simulink model "HandExosThumbRAL_EMG"  (R2013a)
settings: Solver=FixedStepDiscrete  StartTime=0.0  StopTime=inf  FixedStep=1/256  RelTol=1e-3
undefined symbols (not defined in the file or in its folder): currentCFG_EMGTest_UB, serial, UB
libraries: etargetslib x6, instrumentlib x6, dspnetwork x2, xpcutilitieslib x1, gUSBamplib x1
settings Model: Creator=mine  LastModifiedBy=BCI-USER

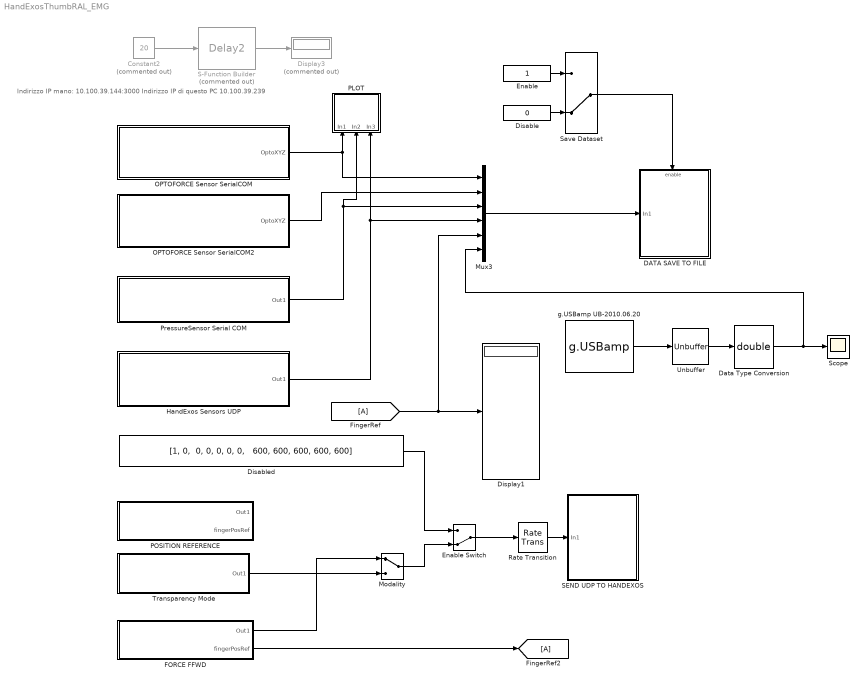
== system HandExosThumbRAL_EMG ==
  note: Indirizzo IP mano: 10.100.39.144:3000
      | Indirizzo IP di questo PC 10.100.39.239
  Constant2 : Constant  Commented=on  Value=20  OutDataTypeStr=uint32  SampleTime=-1
  DATA SAVE TO FILE : Subsystem  TreatAsAtomicUnit=on
  Data Type Conversion : DataTypeConversion  OutDataTypeStr=double
  Disable : Constant  Value=0  OutDataTypeStr=double  SampleTime=-1
  Disabled : Constant  Value="[1, 0,  0, 0, 0, 0, 0,   600, 600, 600, 600, 600]"  OutDataTypeStr=double  SampleTime=-1
  Display1 : Display
  Display3 : Display  Commented=on
  Enable : Constant  OutDataTypeStr=double  SampleTime=-1
  Enable Switch : ManualSwitch  CurrentSetting=0
  FORCE FFWD : Subsystem
  HandExos Sensors UDP : Subsystem
  "Modality " : ManualSwitch
  Mux3 : Mux  Inputs=6
  OPTOFORCE Sensor SerialCOM : Subsystem
  OPTOFORCE Sensor SerialCOM2 : Subsystem
  PLOT : Subsystem
  POSITION REFERENCE : Subsystem
  PressureSensor Serial COM : Subsystem
  Rate Transition : RateTransition
  S-Function Builder : S-Function  Commented=on  InitFcn=try, set_param(gcb,'FunctionName','Delay2'), end  FunctionName=Delay2  SFunctionModules=Delay2_wrapper  EnableBusSupport=off  mask(S-Function Builder){}
      mask help: Simulink:masks:SFunctionBuilder_MD
      mask init:
      | val = [[.9  0.75 0.75 1 1 .9 .9 1]',[1 1 0.75 0.75 .9 .9 1 .9]'];try , sys = get_param(gcb,'SfunBuilderFcnName');if isempty(sys), sys = get_param(gcb,'FunctionName'); end,catch, sys = get_param(gcb,'FunctionName'); end
      settings: CopyFcn=set_param(gcbh,'LinkStatus','none')  PreSaveFcn=try, set_param(gcb,'FunctionName','Delay2'), end  OpenFcn=sfunctionwizard(gcbh)
      mask Display: plot(val(:,1),val(:,2)),disp(sys), port_label('input',1,'u0'), port_label('output',1,'y0')
  SEND UDP TO HANDEXOS : Subsystem  TreatAsAtomicUnit=on  SystemSampleTime=4/256
  Save Dataset : ManualSwitch  CurrentSetting=0
  Scope : Scope
      settings: TimeRange=8  YMin=-225  YMax=200  SaveName=ScopeData3
  Transparency Mode : Subsystem
  Unbuffer : Unbuffer  SampleBasedProcessing=Same as frame based
  g.USBamp UB-2010.06.20 : gUSBamplib/g.USBamp  cfg=currentCFG_EMGTest_UB-2010.06.20.cfg  snr=UB-2010.06.20
  wires:
  Constant2/1 -> S-Function Builder/1
  S-Function Builder/1 -> Display3/1
  Disabled/1 -> Enable Switch/1
  Disable/1 -> Save Dataset/2
  Enable/1 -> Save Dataset/1
  Save Dataset/1 -> DATA SAVE TO FILE/Enable
  OPTOFORCE Sensor SerialCOM/1(OptoXYZ) -> PLOT/1(In1), Mux3/1
  Mux3/1 -> DATA SAVE TO FILE/1(In1)
  Transparency Mode/1(Out1) -> "Modality "/2
  Enable Switch/1 -> Rate Transition/1
  HandExos Sensors UDP/1(Out1) -> Mux3/4, PLOT/3(In3)
  [A] -> Mux3/5, Display1/1
  PressureSensor Serial COM/1(Out1) -> PLOT/2(In2), Mux3/3
  "Modality "/1 -> Enable Switch/2
  OPTOFORCE Sensor SerialCOM2/1(OptoXYZ) -> Mux3/2
  FORCE FFWD/1(Out1) -> "Modality "/1
  FORCE FFWD/2(fingerPosRef) -> [A]
  g.USBamp UB-2010.06.20/1 -> Unbuffer/1
  Unbuffer/1 -> Data Type Conversion/1
  Rate Transition/1 -> SEND UDP TO HANDEXOS/1(In1)
  Data Type Conversion/1 -> Mux3/6, Scope/1

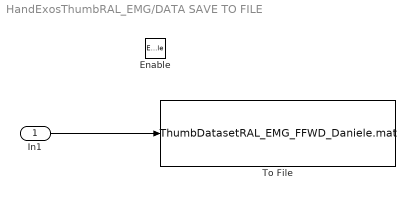
== system HandExosThumbRAL_EMG/DATA SAVE TO FILE ==
  In1 : Inport
  Enable : EnablePort
  To File : ToFile  Filename=ThumbDatasetRAL_EMG_FFWD_Daniele.mat  MatrixName=data
  wires:
  In1/1 -> To File/1

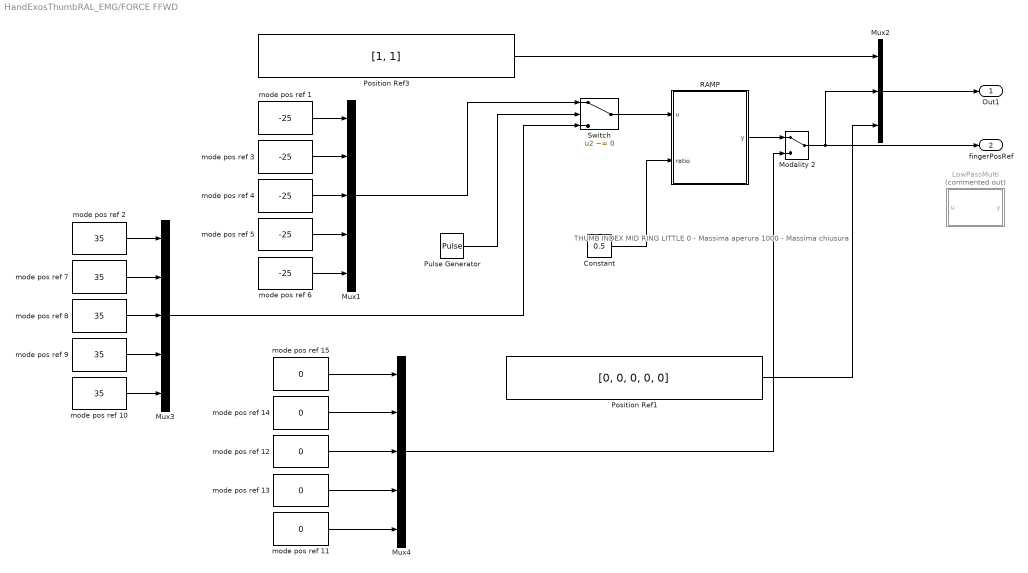
== system HandExosThumbRAL_EMG/FORCE FFWD ==
  note: THUMB
      | INDEX
      | MID
      | RING
      | LITTLE
      |
      | 0 - Massima aperura
      | 1000 - Massima chiusura
  Constant : Constant  Value=0.5
  LowPassMulti : MATLAB Function  Commented=on  TreatAsAtomicUnit=on
  Modality 2 : ManualSwitch
  Mux1 : Mux  Inputs=5
  Mux2 : Mux  Inputs=3
  Mux3 : Mux  Inputs=5
  Mux4 : Mux  Inputs=5
  Position Ref1 : Constant  Value=[0, 0, 0, 0, 0]  OutDataTypeStr=double  SampleTime=-1
  Position Ref3 : Constant  Value=[1, 1]  OutDataTypeStr=double  SampleTime=-1
  Pulse Generator : DiscretePulseGenerator  PulseType=Time based  Period=10  PulseWidth=50
  RAMP : MATLAB Function  TreatAsAtomicUnit=on
  Switch : Switch  Criteria=u2 ~= 0
  mode pos ref {1,3..6} (5 alike) : Constant  Value=-25  OutDataTypeStr=double  SampleTime=-1
  mode pos ref {2,7..10} (5 alike) : Constant  Value=35  OutDataTypeStr=double  SampleTime=-1
  mode pos ref {11..15} (5 alike) : Constant  Value=0  OutDataTypeStr=double  SampleTime=-1
  Out1 : Outport
  fingerPosRef : Outport  Port=2
  wires:
  Mux2/1 -> Out1/1
  mode pos ref 1/1 -> Mux1/1
  mode pos ref 6/1 -> Mux1/5
  mode pos ref 5/1 -> Mux1/4
  mode pos ref 4/1 -> Mux1/3
  mode pos ref 3/1 -> Mux1/2
  Position Ref3/1 -> Mux2/1
  mode pos ref 10/1 -> Mux3/5
  mode pos ref 9/1 -> Mux3/4
  mode pos ref 8/1 -> Mux3/3
  mode pos ref 7/1 -> Mux3/2
  mode pos ref 2/1 -> Mux3/1
  mode pos ref 14/1 -> Mux4/2
  mode pos ref 13/1 -> Mux4/4
  mode pos ref 12/1 -> Mux4/3
  mode pos ref 11/1 -> Mux4/5
  Constant/1 -> RAMP/2(ratio)
  Mux1/1 -> Switch/1
  Mux3/1 -> Switch/3
  Pulse Generator/1 -> Switch/2
  mode pos ref 15/1 -> Mux4/1
  RAMP/1(y) -> Modality 2/1
  Modality 2/1 -> Mux2/2, fingerPosRef/1
  Mux4/1 -> Modality 2/2
  Switch/1 -> RAMP/1(u)
  Position Ref1/1 -> Mux2/3

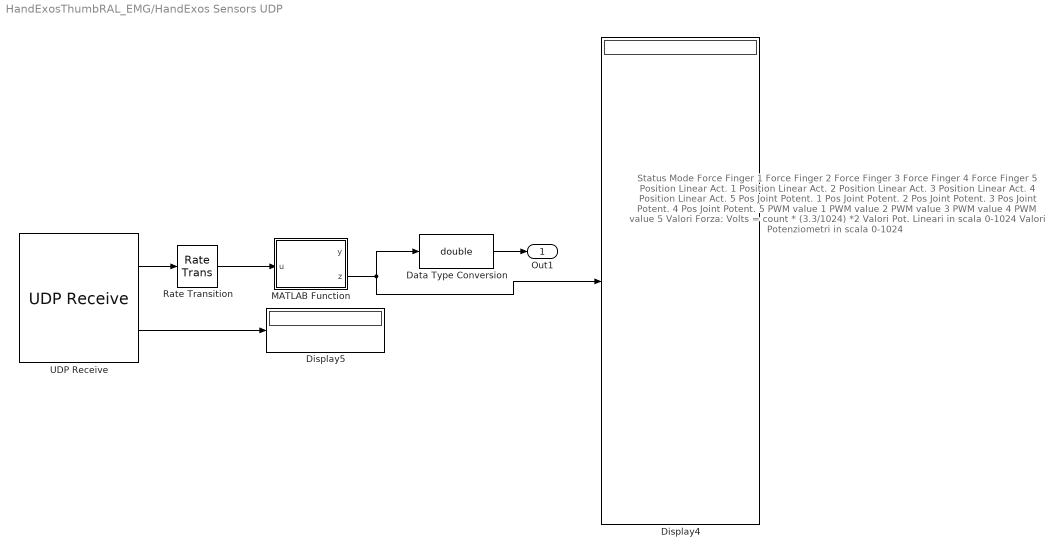
== system HandExosThumbRAL_EMG/HandExos Sensors UDP ==
  note: Status
      | Mode
      | Force Finger 1
      | Force Finger 2
      | Force Finger 3
      | Force Finger 4
      | Force Finger 5
      | Position Linear Act. 1
      | Position Linear Act. 2
      | Position Linear Act. 3
      | Position Linear Act. 4
      | Position Linear Act. 5
      | Pos Joint Potent. 1
      | Pos Joint Potent. 2
      | Pos Joint Potent. 3
      | Pos Joint Potent. 4
      | Pos Joint Potent. 5
      | PWM value 1
      | PWM value 2
      | PWM value 3
      | PWM value 4
      | PWM value 5
      |
      | Valori Forza:    Volts = count * (3.3/1024) *2
      | Valori Pot. Lineari in scala 0-1024
      | Valori Potenziometri in scala 0-1024
  Data Type Conversion : DataTypeConversion  OutDataTypeStr=double
  Display4 : Display
  Display5 : Display
  MATLAB Function : MATLAB Function  TreatAsAtomicUnit=on
  Rate Transition : RateTransition
  UDP Receive : dspnetwork/UDP Receive  localURL='0.0.0.0'  localPort=12001  remoteURL='10.100.39.144'  remotePort=-1  recvBufferSize=73  dims=22  signalDatatype=single  isVarSize=off  showBlockingTime=off  blockingTime=0  sampletime=4/256
  Out1 : Outport
  wires:
  MATLAB Function/2(z) -> Data Type Conversion/1, Display4/1
  UDP Receive/1 -> Rate Transition/1
  UDP Receive/2 -> Display5/1
  Data Type Conversion/1 -> Out1/1
  Rate Transition/1 -> MATLAB Function/1(u)

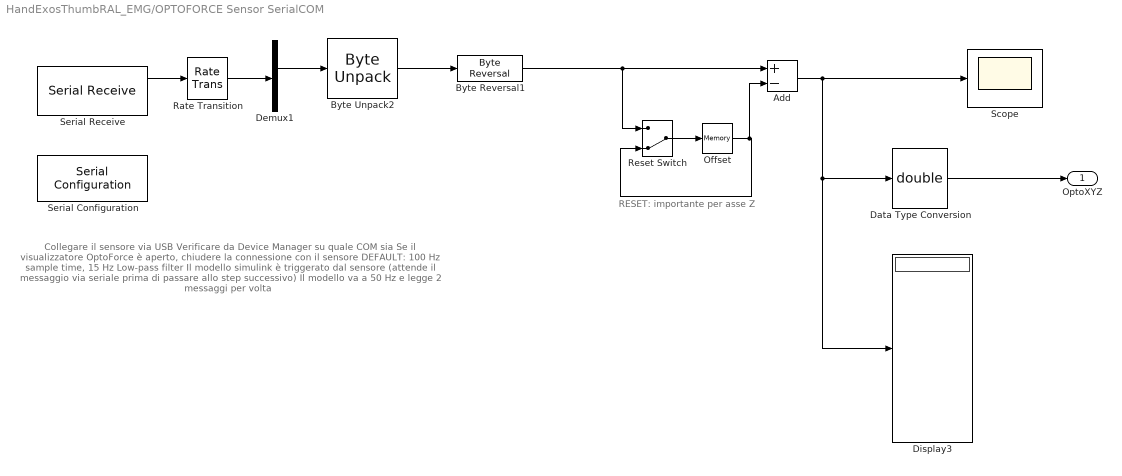
== system HandExosThumbRAL_EMG/OPTOFORCE Sensor SerialCOM ==
  note: RESET: importante per asse Z
  note: Collegare il sensore via USB
      | Verificare da Device Manager su quale COM sia
      | Se il visualizzatore OptoForce è aperto, chiudere la connessione con il sensore
      |
      | DEFAULT: 100 Hz sample time, 15 Hz Low-pass filter
      |
      | Il modello simulink è triggerato dal sensore
      | (attende il messaggio via seriale prima di passare allo step successivo)
      | Il modello va a 50 Hz e legge 2 messaggi per volta
  Add : Sum  Inputs=+-
  Byte Reversal1 : etargetslib/Byte Reversal  numInp=1
  Byte Unpack2 : etargetslib/Byte Unpack  dimensions={3}  datatypes={'int16'}  byteAlign=1
  Data Type Conversion : DataTypeConversion  OutDataTypeStr=double
  Demux1 : Demux  Outputs="[3 6 20  29]"
  Display3 : Display
  Offset : Memory  X0=[0 0 32460]
  Rate Transition : RateTransition
  Reset Switch : ManualSwitch  CurrentSetting=0
  Scope : Scope
      settings: YMin=-800  YMax=1100
  Serial Configuration : instrumentlib/Serial Configuration  Priority=-200000  ComPortMenu=<Please select a port...>  ComPort=COM14  ObjConstructor=serial('COM14');  BaudRate=115200  DataBits=8  Parity=none  StopBits=1  FlowControl=none  Timeout=5  ByteOrder=LittleEndian
  Serial Receive : instrumentlib/Serial Receive  ComPortMenu=COM14  ComPort=COM14  ObjConstructor=serial('COM14');  Terminator=<none>  DataSize="[58   1]"  DataType=uint8  EnableBlockingMode=off  ActionDataUnavailable=Output last received value  CustomValue=0  SampleTime=4/256
  OptoXYZ : Outport
  wires:
  Demux1/2 -> Byte Unpack2/1
  Byte Unpack2/1 -> Byte Reversal1/1
  Reset Switch/1 -> Offset/1
  Offset/1 -> Reset Switch/2, Add/2
  Serial Receive/1 -> Rate Transition/1
  Data Type Conversion/1 -> OptoXYZ/1
  Add/1 -> Display3/1, Data Type Conversion/1, Scope/1
  Byte Reversal1/1 -> Reset Switch/1, Add/1
  Rate Transition/1 -> Demux1/1

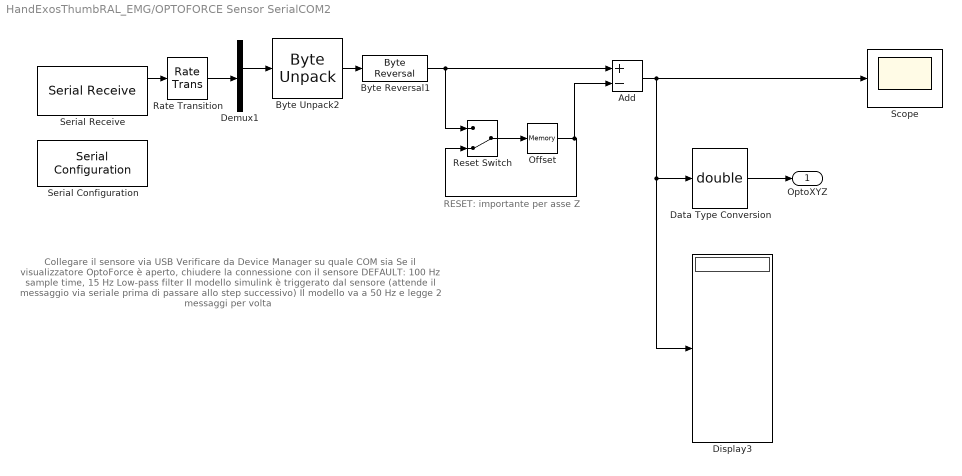
== system HandExosThumbRAL_EMG/OPTOFORCE Sensor SerialCOM2 ==
  note: RESET: importante per asse Z
  note: Collegare il sensore via USB
      | Verificare da Device Manager su quale COM sia
      | Se il visualizzatore OptoForce è aperto, chiudere la connessione con il sensore
      |
      | DEFAULT: 100 Hz sample time, 15 Hz Low-pass filter
      |
      | Il modello simulink è triggerato dal sensore
      | (attende il messaggio via seriale prima di passare allo step successivo)
      | Il modello va a 50 Hz e legge 2 messaggi per volta
  Add : Sum  Inputs=+-
  Byte Reversal1 : etargetslib/Byte Reversal  numInp=1
  Byte Unpack2 : etargetslib/Byte Unpack  dimensions={3}  datatypes={'int16'}  byteAlign=1
  Data Type Conversion : DataTypeConversion  OutDataTypeStr=double
  Demux1 : Demux  Outputs="[3 6 20  29]"
  Display3 : Display
  Offset : Memory  X0=[0 0 32460]
  Rate Transition : RateTransition
  Reset Switch : ManualSwitch  CurrentSetting=0
  Scope : Scope
      settings: YMin=-300  YMax=1200
  Serial Configuration : instrumentlib/Serial Configuration  Priority=-200000  ComPortMenu=COM24  ComPort=COM24  ObjConstructor=serial('COM24');  BaudRate=115200  DataBits=8  Parity=none  StopBits=1  FlowControl=none  Timeout=5  ByteOrder=LittleEndian
  Serial Receive : instrumentlib/Serial Receive  ComPortMenu=COM24  ComPort=COM24  ObjConstructor=serial('COM24');  Terminator=<none>  DataSize="[58   1]"  DataType=uint8  EnableBlockingMode=off  ActionDataUnavailable=Output last received value  CustomValue=0  SampleTime=4/256
  OptoXYZ : Outport
  wires:
  Demux1/2 -> Byte Unpack2/1
  Byte Reversal1/1 -> Reset Switch/1, Add/1
  Byte Unpack2/1 -> Byte Reversal1/1
  Reset Switch/1 -> Offset/1
  Add/1 -> Display3/1, Data Type Conversion/1, Scope/1
  Serial Receive/1 -> Rate Transition/1
  Offset/1 -> Reset Switch/2, Add/2
  Data Type Conversion/1 -> OptoXYZ/1
  Rate Transition/1 -> Demux1/1

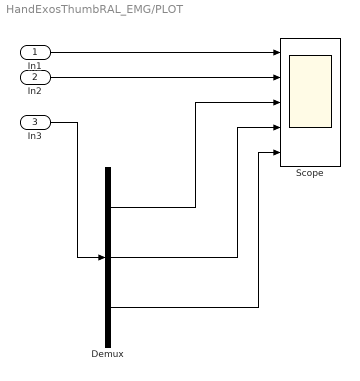
== system HandExosThumbRAL_EMG/PLOT ==
  In1 : Inport
  In2 : Inport  Port=2
  In3 : Inport  Port=3
  Demux : Demux  Outputs=[2 1 4 1 9 1 4]
  Scope : Scope  NumInputPorts=5
      settings: YMin=-1000~237000~32.5~0~-30  YMax=5000~244000~60~350~40  SaveName=ScopeData2
  wires:
  In1/1 -> Scope/1
  In2/1 -> Scope/2
  In3/1 -> Demux/1
  Demux/2 -> Scope/3
  Demux/4 -> Scope/4
  Demux/6 -> Scope/5

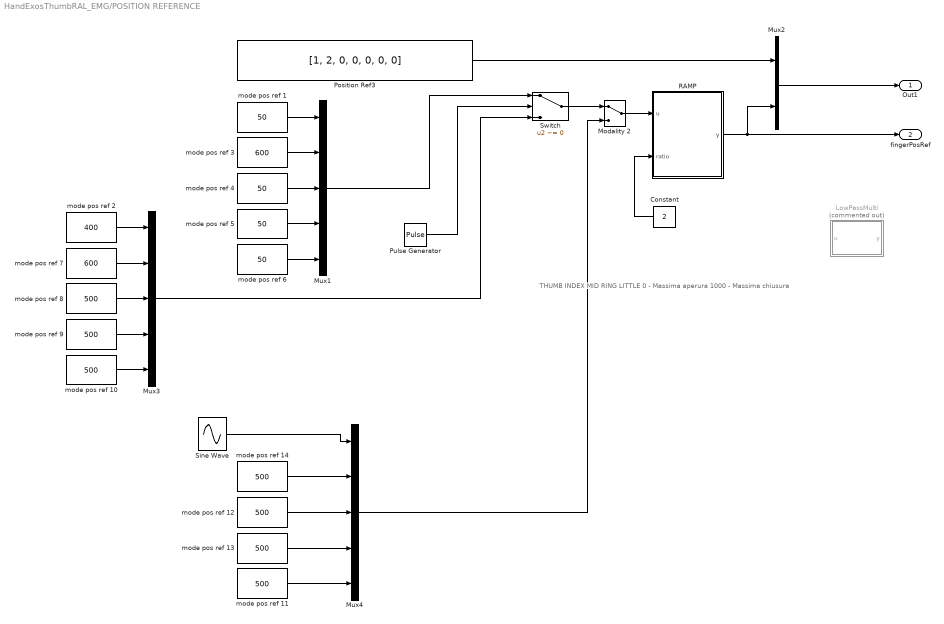
== system HandExosThumbRAL_EMG/POSITION REFERENCE ==
  note: THUMB
      | INDEX
      | MID
      | RING
      | LITTLE
      |
      | 0 - Massima aperura
      | 1000 - Massima chiusura
  Constant : Constant  Value=2
  LowPassMulti : MATLAB Function  Commented=on  TreatAsAtomicUnit=on
  Modality 2 : ManualSwitch
  Mux1 : Mux  Inputs=5
  Mux2 : Mux  Inputs=2
  Mux3 : Mux  Inputs=5
  Mux4 : Mux  Inputs=5
  Position Ref3 : Constant  Value=[1, 2, 0, 0, 0, 0, 0]  OutDataTypeStr=double  SampleTime=-1
  Pulse Generator : DiscretePulseGenerator  PulseType=Time based  Period=10  PulseWidth=50
  RAMP : MATLAB Function  TreatAsAtomicUnit=on
  Sine Wave : Sin  Amplitude=200  Bias=300  Frequency=2*pi/10  SampleTime=0
  Switch : Switch  Criteria=u2 ~= 0
  mode pos ref {1,4..6} (4 alike) : Constant  Value=50  OutDataTypeStr=double  SampleTime=-1
  mode pos ref {8..14} (7 alike) : Constant  Value=500  OutDataTypeStr=double  SampleTime=-1
  mode pos ref 2 : Constant  Value=400  OutDataTypeStr=double  SampleTime=-1
  mode pos ref 3 : Constant  Value=600  OutDataTypeStr=double  SampleTime=-1
  mode pos ref 7 : Constant  Value=600  OutDataTypeStr=double  SampleTime=-1
  Out1 : Outport
  fingerPosRef : Outport  Port=2
  wires:
  Mux2/1 -> Out1/1
  mode pos ref 1/1 -> Mux1/1
  mode pos ref 6/1 -> Mux1/5
  mode pos ref 5/1 -> Mux1/4
  mode pos ref 4/1 -> Mux1/3
  mode pos ref 3/1 -> Mux1/2
  Position Ref3/1 -> Mux2/1
  mode pos ref 10/1 -> Mux3/5
  mode pos ref 9/1 -> Mux3/4
  mode pos ref 8/1 -> Mux3/3
  mode pos ref 7/1 -> Mux3/2
  mode pos ref 2/1 -> Mux3/1
  Sine Wave/1 -> Mux4/1
  mode pos ref 14/1 -> Mux4/2
  mode pos ref 13/1 -> Mux4/4
  mode pos ref 12/1 -> Mux4/3
  mode pos ref 11/1 -> Mux4/5
  Switch/1 -> Modality 2/1
  Modality 2/1 -> RAMP/1(u)
  Mux4/1 -> Modality 2/2
  Constant/1 -> RAMP/2(ratio)
  RAMP/1(y) -> Mux2/2, fingerPosRef/1
  Mux1/1 -> Switch/1
  Mux3/1 -> Switch/3
  Pulse Generator/1 -> Switch/2

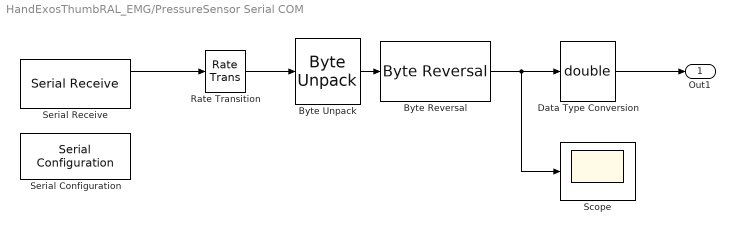
== system HandExosThumbRAL_EMG/PressureSensor Serial COM ==
  Byte Reversal : etargetslib/Byte Reversal  numInp=1
  Byte Unpack : etargetslib/Byte Unpack  dimensions={[1]}  datatypes={'int32'}  byteAlign=1
  Data Type Conversion : DataTypeConversion  OutDataTypeStr=double
  Rate Transition : RateTransition
  Scope : Scope
      settings: YMin=237750  YMax=242250
  Serial Configuration : instrumentlib/Serial Configuration  Priority=-200000  ComPortMenu=<Please select a port...>  ComPort=COM23  ObjConstructor=serial('COM23');  BaudRate=115200  DataBits=8  Parity=none  StopBits=1  FlowControl=none  Timeout=5  ByteOrder=LittleEndian
  Serial Receive : instrumentlib/Serial Receive  ComPortMenu=COM23  ComPort=COM23  ObjConstructor=serial('COM23');  Terminator=<none>  DataSize="[4  1]"  DataType=uint8  EnableBlockingMode=off  ActionDataUnavailable=Output last received value  CustomValue=0  SampleTime=4/256
  Out1 : Outport
  wires:
  Serial Receive/1 -> Rate Transition/1
  Byte Unpack/1 -> Byte Reversal/1
  Byte Reversal/1 -> Scope/1, Data Type Conversion/1
  Data Type Conversion/1 -> Out1/1
  Rate Transition/1 -> Byte Unpack/1

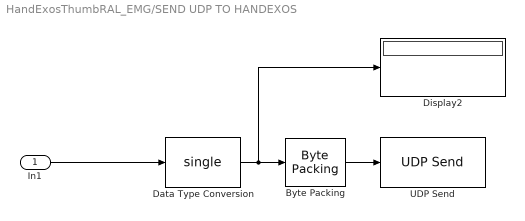
== system HandExosThumbRAL_EMG/SEND UDP TO HANDEXOS ==
  In1 : Inport
  "Byte Packing " : xpcutilitieslib/Byte Packing   MaskPackedDataType=uint8  MaskUnpackedDataTypes={'single'}  MaskAlignment=1
  Data Type Conversion : DataTypeConversion  OutDataTypeStr=single
  Display2 : Display
  UDP Send : dspnetwork/UDP Send  remoteURL='10.100.39.144'  remotePort=12000  localURL='0.0.0.0'  localPortSource=Automatically determine  localPort=-1  sampletime=-1  separateLengthPort=0
  wires:
  Data Type Conversion/1 -> Display2/1, "Byte Packing "/1
  "Byte Packing "/1 -> UDP Send/1
  In1/1 -> Data Type Conversion/1

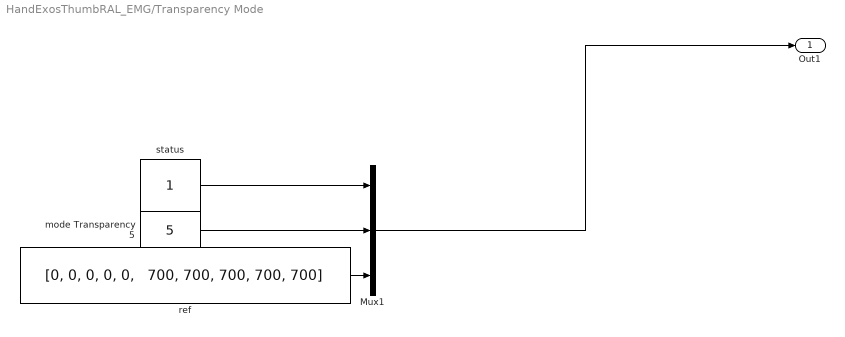
== system HandExosThumbRAL_EMG/Transparency Mode ==
  Mux1 : Mux  Inputs=[1 1 10]
  mode Transparency 5 : Constant  Value=5  OutDataTypeStr=double  SampleTime=-1
  ref : Constant  Value="[0, 0, 0, 0, 0,   700, 700, 700, 700, 700]"  OutDataTypeStr=double  SampleTime=-1
  status : Constant  OutDataTypeStr=double  SampleTime=-1
  Out1 : Outport
  wires:
  Mux1/1 -> Out1/1
  status/1 -> Mux1/1
  mode Transparency 5/1 -> Mux1/2
  ref/1 -> Mux1/3

== matlab function HandExosThumbRAL_EMG/HandExos Sensors UDP/MATLAB Function ==
  data: u input; y output; z output
function [y,z] = fcn(u)
%#codegen
persistent old_values

if(isempty(old_values))
    old_values = single(zeros(22,1));
end

if ((u(1)==0.0) && (u(2)==0.0))
    y = old_values;
else
    y = u;
    old_values = u;
end

z = old_values;
    


y = u;

== matlab function HandExosThumbRAL_EMG/POSITION REFERENCE/RAMP ==
  data: u input; y output; ratio input
function y = fcn(u, ratio)
%#codegen

persistent y_old;

if(isempty(y_old))
    y_old = zeros(1,5);
end

y = zeros(1,5); 

for i=1:1:5
    
    delta = u(i)-y_old(i);
    if(delta>=0)
        if(delta > ratio)
            y(i) = y_old(i) + ratio;
        else
             y(i) = u(i);           
        end
    else
        if(delta < -ratio)
            y(i) = y_old(i)-ratio;
        else
            y(i) = u(i);
        end
    end
        
    y_old(i) = y(i);
    
end

== matlab function HandExosThumbRAL_EMG/FORCE FFWD/LowPassMulti ==
  data: u input; y output
function y = fcn(u)
%#codegen

persistent old_y;
if(isempty(old_y))
    old_y = zeros(1,5);
end

ts = 0.02;
tf = 0.5;
b = ts/(ts+tf);
a = tf/(ts+tf);

y = zeros(1,5); 

for i=1:1:5
    
    y(i) = old_y(i)*a + u(i)*b;
    old_y(i) = y(i);
    
end

== matlab function HandExosThumbRAL_EMG/FORCE FFWD/RAMP ==
  data: u input; y output; ratio input
function y = fcn(u, ratio)
%#codegen

persistent y_old;

if(isempty(y_old))
    y_old = zeros(1,5);
end

y = zeros(1,5); 

for i=1:1:5
    
    delta = u(i)-y_old(i);
    if(delta>=0)
        if(delta > ratio)
            y(i) = y_old(i) + ratio;
        else
             y(i) = u(i);           
        end
    else
        if(delta < -ratio)
            y(i) = y_old(i)-ratio;
        else
            y(i) = u(i);
        end
    end
        
    y_old(i) = y(i);
    
end

== matlab function HandExosThumbRAL_EMG/POSITION REFERENCE/LowPassMulti ==
  data: u input; y output
function y = fcn(u)
%#codegen

persistent old_y;
if(isempty(old_y))
    old_y = zeros(1,5);
end

ts = 0.02;
tf = 0.5;
b = ts/(ts+tf);
a = tf/(ts+tf);

y = zeros(1,5); 

for i=1:1:5
    
    y(i) = old_y(i)*a + u(i)*b;
    old_y(i) = y(i);
    
end
